simulink model "part4b"  (R2018a)
settings: Solver=VariableStepAuto  StartTime=0.0  StopTime=40000  RelTol=1e-3
values from neighbouring files (symbols this model uses):
  ain = 90    [variables.m]
  aout = 0    [variables.m]
  c = 16    [variables.m]
  kout = 0.1587    [variables.m]
  qin = 10*.134/60    (= 0.0223333333333)    [variables.m]
settings Model: Creator=jschm  LastModifiedBy=jschm

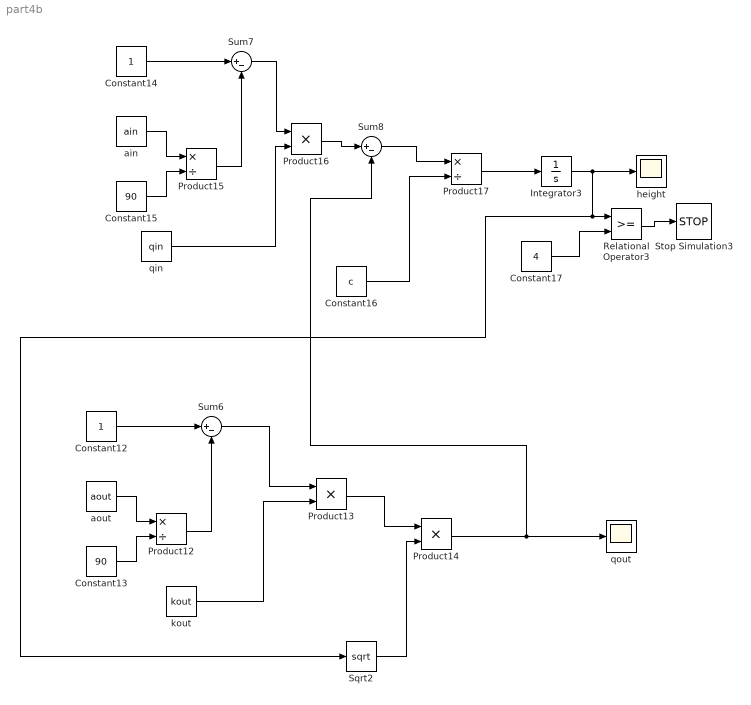
== system part4b ==
  Constant12 : Constant
  Constant13 : Constant  Value=90
  Constant14 : Constant
  Constant15 : Constant  Value=90
  Constant16 : Constant  Value=c
  Constant17 : Constant  Value=4
  Integrator3 : Integrator
  Product12 : Product  Inputs=*/
  Product13 : Product
  Product14 : Product
  Product15 : Product  Inputs=*/
  Product16 : Product
  Product17 : Product  Inputs=*/
  Relational Operator3 : RelationalOperator  OutDataTypeStr=boolean  RndMeth=Simplest
  Sqrt2 : Sqrt  SaturateOnIntegerOverflow=on
  Stop Simulation3 : Stop
  Sum6 : Sum  Inputs=|+-
  Sum7 : Sum  Inputs=|+-
  Sum8 : Sum  Inputs=|+-
  ain : Constant  Value=ain
  aout : Constant  Value=aout
  height : Scope
  kout : Constant  Value=kout
  qin : Constant  Value=qin
  qout : Scope
  wires:
  Sum8/1 -> Product17/1
  Product14/1 -> Sum8/2, qout/1
  Product17/1 -> Integrator3/1
  Constant15/1 -> Product15/2
  Constant17/1 -> Relational Operator3/2
  Sum7/1 -> Product16/1
  ain/1 -> Product15/1
  Product16/1 -> Sum8/1
  Integrator3/1 -> Sqrt2/1, Relational Operator3/1, height/1
  Constant16/1 -> Product17/2
  Constant14/1 -> Sum7/1
  Relational Operator3/1 -> Stop Simulation3/1
  Product15/1 -> Sum7/2
  Constant12/1 -> Sum6/1
  Sqrt2/1 -> Product14/2
  Sum6/1 -> Product13/1
  Product13/1 -> Product14/1
  Constant13/1 -> Product12/2
  aout/1 -> Product12/1
  kout/1 -> Product13/2
  Product12/1 -> Sum6/2
  qin/1 -> Product16/2
